simulink model "turbulence"  (R2020b)
settings: Solver=VariableStepAuto  StartTime=0.0  StopTime=100  RelTol=1e-3
undefined symbols (not defined in the file): F, Light, MIL
libraries: simulink_extras x2, aerolibwind2 x1
settings Model: Creator=ben  LastModifiedBy=ben

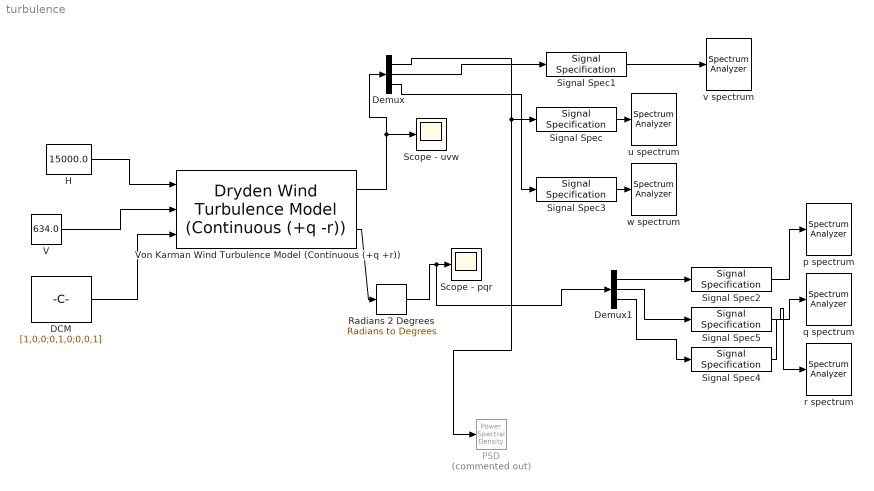
== system turbulence ==
  DCM : Constant  Value=[1,0,0;0,1,0;0,0,1]
  Demux : Demux  Outputs=3
  Demux1 : Demux  Outputs=3
  H : Constant  Value=15000.0
  PSD : simulink_extras/Additional Sinks/Power Spectral Density  Commented=on  npts=128  fftpts=512  HowOften=64  sampleT=0.1
      settings: SourceProductBaseCode=SL
  Radians 2 Degrees : simulink_extras/Transformations/Radians to Degrees
  Scope - pqr : Scope
  Scope - uvw : Scope
  Signal Spec{,1..5} (6 alike) : SignalSpecification  SampleTime=0.01
  V : Constant  Value=634.0
  Von Karman Wind Turbulence Model (Continuous (+q +r)) : aerolibwind2/Dryden Wind Turbulence Model  (Continuous (+q -r))  units=English (Velocity in ft/s)  spec=MIL-F-8785C  model=Continuous Von Karman (+q +r)  W20=15  Wdeg=0  TurbProb=10^-2 - Light  L_high=1500  Wingspan=30  ts=0.01  Seed=[23341 23342 23343 23344]  T_on=on
  p spectrum : SpectrumAnalyzer
  q spectrum : SpectrumAnalyzer
  r spectrum : SpectrumAnalyzer
  u spectrum : SpectrumAnalyzer
  v spectrum : SpectrumAnalyzer
  w spectrum : SpectrumAnalyzer
  wires:
  Von Karman Wind Turbulence Model (Continuous (+q +r))/1 -> Demux/1, Scope - uvw/1
  V/1 -> Von Karman Wind Turbulence Model (Continuous (+q +r))/2
  DCM/1 -> Von Karman Wind Turbulence Model (Continuous (+q +r))/3
  H/1 -> Von Karman Wind Turbulence Model (Continuous (+q +r))/1
  Von Karman Wind Turbulence Model (Continuous (+q +r))/2 -> Radians 2 Degrees/1
  Radians 2 Degrees/1 -> Demux1/1, Scope - pqr/1
  Demux/3 -> Signal Spec3/1
  Demux/2 -> Signal Spec1/1
  Demux/1 -> PSD/1, Signal Spec/1
  Signal Spec/1 -> u spectrum/1
  Signal Spec1/1 -> v spectrum/1
  Demux1/3 -> Signal Spec4/1
  Demux1/2 -> Signal Spec5/1
  Signal Spec2/1 -> p spectrum/1
  Demux1/1 -> Signal Spec2/1
  Signal Spec3/1 -> w spectrum/1
  Signal Spec4/1 -> q spectrum/1
  Signal Spec5/1 -> r spectrum/1
